simulink model "rtwdemo_paramdt"  (Simulink 7.6)
settings: Solver=FixedStepDiscrete  StartTime=0.0  StopTime=10.0  RelTol=1e-3  SampleTimeConstraint=STIndependent
PostLoadFcn:
  | rtwdemo_paramdt_data
undefined symbols (not defined in the file or in its folder): Kalias, Kcs, Kfixpt, Kinline, Kint8, Ksingle, Kuser
libraries: rtwdemowidgets x3
Description:
  | Controlling the Data Types of Tunable Parameters
settings Model: Creator=The MathWorks Inc.  CovMetricSettings=d  ExtModeAutoUpdateStatusClock=off  TunableVars=Kcs,Kint8,Ksingle  TunableVarsStorageClass=ExportedGlobal,ExportedGlobal,ExportedGlobal  TunableVarsTypeQualifier=,,
settings DataIOCC: SaveOutput=off  SaveTime=off  SignalLoggingName=sigsOut
settings OptimizationCC: InlineParams=on  InlineInvariantSignals=on  StateBitsets=on  DataBitsets=on  UseTempVars=on  EfficientFloat2IntCast=on  EfficientMapNaN2IntZero=off
settings DebuggingCC: CheckExecutionContextPreStartOutputMsg=on  CheckExecutionContextRuntimeOutputMsg=on  SolverPrmCheckMsg=none  ParameterDowncastMsg=none  ParameterOverflowMsg=none  ParameterPrecisionLossMsg=none  StrictBusMsg=ErrorOnBusTreatedAsVector
settings HardwareCC: ProdIntDivRoundTo=Zero  ProdEndianess=LittleEndian  ProdHWDeviceType=Generic->32-bit Embedded Processor  TargetIntDivRoundTo=Zero  TargetEndianess=LittleEndian  TargetHWDeviceType=Generic->MATLAB Host Computer  ProdEqTarget=off
settings SFSimCC: SimParseCustomCode=off
settings RTWCC: TLCOptions=-p0  GenerateReport=on  RTWVerbose=off  ProcessScript=grt_make_rtw_hook  LaunchReport=on
settings CodeAppCC: ForceParamTrailComments=on
settings GRTTargetCC: TargetFcnLib=ansi_tfl_tmw.mat

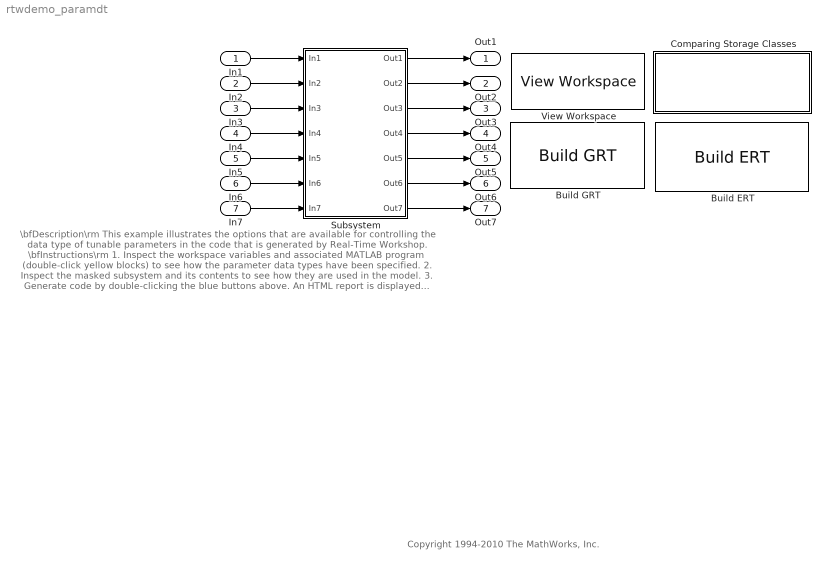
== system rtwdemo_paramdt ==
  note: \bfDescription\rm
      | This example illustrates the options that are available for controlling the data type of
      | tunable parameters in the code that is generated by Real-Time Workshop.
      |
      | \bfInstructions\rm
      | 1. Inspect the workspace variables and associated MATLAB program (double-click yellow blocks)
      |     to see how the parameter data types have been specified.
      | 2. Inspect the masked subsystem and its contents to see how they are used in the model.
      | 3. Generate code by double-clicking the blue buttons above.
      |     An HTML report is displayed automatically.
      | 4. Inspect the generated source files and take note of
      |     - The data types used in the parameter declarations/definitions
      |     - How the parameters are used in the code for the Gain and Saturation blocks
      |
      | \bfNote\rm
      | Inline parameters and storage classes must be selected to preserve parameter
      | identifiers in the generated code.
  note: Copyright 1994-2010 The MathWorks, Inc.
  In1 : Inport  OutDataTypeStr=single  PortDimensions=1
  In2 : Inport  Port=2  OutDataTypeStr=single  PortDimensions=1
  In3 : Inport  Port=3  OutDataTypeStr=single  PortDimensions=1
  In4 : Inport  Port=4  OutDataTypeStr=single  PortDimensions=1
  In5 : Inport  Port=5  OutDataTypeStr=single  PortDimensions=1
  In6 : Inport  Port=6  OutDataTypeStr=single  PortDimensions=1
  In7 : Inport  Port=7  OutDataTypeStr=single  PortDimensions=1
  Build ERT : rtwdemowidgets/Build ERT  SystemSampleTime=-1  attrib_overrides={}
  Build GRT : rtwdemowidgets/Build GRT  SystemSampleTime=-1  attrib_overrides={}
  Comparing Storage Classes : Subsystem
      settings: OpenFcn=edit rtwdemo_paramdt_data.m
      mask Display: disp(['View MATLAB program For\nCreating Variables\n(double-click)']);
  Subsystem : Subsystem
  View Workspace : rtwdemowidgets/View Workspace  SystemSampleTime=-1
  Out1 : Outport
  Out2 : Outport  Port=2
  Out3 : Outport  Port=3
  Out4 : Outport  Port=4
  Out5 : Outport  Port=5
  Out6 : Outport  Port=6
  Out7 : Outport  Port=7
  wires:
  In1/1 -> Subsystem/1(In1)
  In2/1 -> Subsystem/2(In2)
  In3/1 -> Subsystem/3(In3)
  In4/1 -> Subsystem/4(In4)
  In5/1 -> Subsystem/5(In5)
  In6/1 -> Subsystem/6(In6)
  In7/1 -> Subsystem/7(In7)
  Subsystem/1(Out1) -> Out1/1
  Subsystem/2(Out2) -> Out2/1
  Subsystem/3(Out3) -> Out3/1
  Subsystem/4(Out4) -> Out4/1
  Subsystem/5(Out5) -> Out5/1
  Subsystem/6(Out6) -> Out6/1
  Subsystem/7(Out7) -> Out7/1

== system rtwdemo_paramdt/Comparing Storage Classes ==

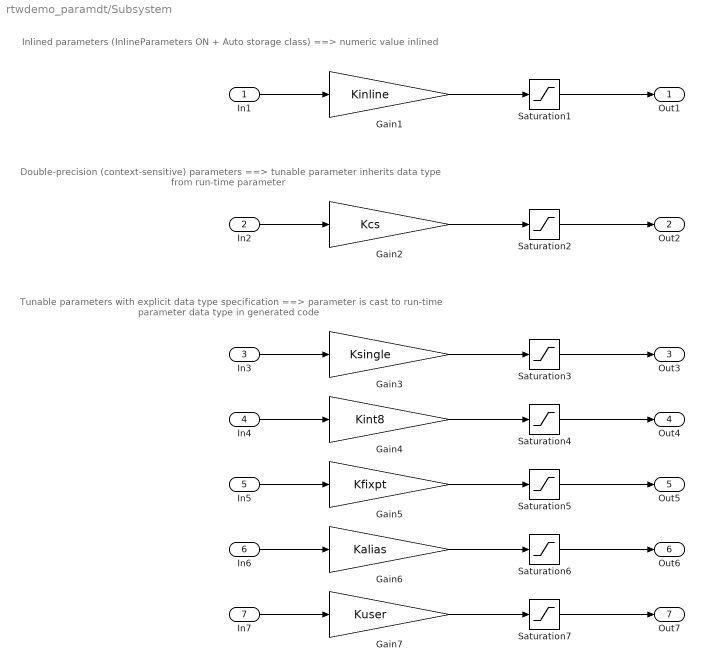
== system rtwdemo_paramdt/Subsystem ==
  note: Double-precision (context-sensitive) parameters
      | ==> tunable parameter inherits data type from run-time parameter
  note: Tunable parameters with explicit data type specification
      | ==> parameter is cast to run-time parameter data type in generated code
  note: Inlined parameters (InlineParameters ON + Auto storage class)
      | ==> numeric value inlined
  In1 : Inport  OutDataTypeStr=single
  In2 : Inport  Port=2  OutDataTypeStr=single
  In3 : Inport  Port=3  OutDataTypeStr=single
  In4 : Inport  Port=4  OutDataTypeStr=single
  In5 : Inport  Port=5  OutDataTypeStr=single
  In6 : Inport  Port=6  OutDataTypeStr=single
  In7 : Inport  Port=7  OutDataTypeStr=single
  Gain1 : Gain  Gain=Kinline  OutDataTypeStr=Inherit: Same as input  ParamDataTypeStr=Inherit: Same as input
  Gain2 : Gain  Gain=Kcs  OutDataTypeStr=Inherit: Same as input  ParamDataTypeStr=Inherit: Same as input
  Gain3 : Gain  Gain=Ksingle  OutDataTypeStr=Inherit: Same as input  ParamDataTypeStr=Inherit: Same as input
  Gain4 : Gain  Gain=Kint8  OutDataTypeStr=Inherit: Same as input  ParamDataTypeStr=Inherit: Same as input
  Gain5 : Gain  Gain=Kfixpt  OutDataTypeStr=Inherit: Same as input  ParamDataTypeStr=Inherit: Same as input
  Gain6 : Gain  Gain=Kalias  OutDataTypeStr=Inherit: Same as input  ParamDataTypeStr=Inherit: Same as input
  Gain7 : Gain  Gain=Kuser  OutDataTypeStr=Inherit: Same as input  ParamDataTypeStr=Inherit: Same as input
  Saturation1 : Saturate  UpperLimit=Kinline  LowerLimit=0
      settings: AttributesFormatString=Upper: %<UpperLimit>\nLower: %<LowerLimit>
  Saturation2 : Saturate  UpperLimit=Kcs  LowerLimit=0
      settings: AttributesFormatString=Upper: %<UpperLimit>\nLower: %<LowerLimit>
  Saturation3 : Saturate  UpperLimit=Ksingle  LowerLimit=0
      settings: AttributesFormatString=Upper: %<UpperLimit>\nLower: %<LowerLimit>
  Saturation4 : Saturate  UpperLimit=Kint8  LowerLimit=0
      settings: AttributesFormatString=Upper: %<UpperLimit>\nLower: %<LowerLimit>
  Saturation5 : Saturate  UpperLimit=Kfixpt  LowerLimit=0
      settings: AttributesFormatString=Upper: %<UpperLimit>\nLower: %<LowerLimit>
  Saturation6 : Saturate  UpperLimit=Kalias  LowerLimit=0
      settings: AttributesFormatString=Upper: %<UpperLimit>\nLower: %<LowerLimit>
  Saturation7 : Saturate  UpperLimit=Kuser  LowerLimit=0
      settings: AttributesFormatString=Upper: %<UpperLimit>\nLower: %<LowerLimit>
  Out1 : Outport
  Out2 : Outport  Port=2
  Out3 : Outport  Port=3
  Out4 : Outport  Port=4
  Out5 : Outport  Port=5
  Out6 : Outport  Port=6
  Out7 : Outport  Port=7
  wires:
  In2/1 -> Gain2/1
  Gain2/1 -> Saturation2/1
  In3/1 -> Gain3/1
  Gain3/1 -> Saturation3/1
  In4/1 -> Gain4/1
  Gain4/1 -> Saturation4/1
  In5/1 -> Gain5/1
  Gain5/1 -> Saturation5/1
  Saturation2/1 -> Out2/1
  Saturation3/1 -> Out3/1
  Saturation4/1 -> Out4/1
  Saturation5/1 -> Out5/1
  In6/1 -> Gain6/1
  Gain6/1 -> Saturation6/1
  Saturation6/1 -> Out6/1
  In7/1 -> Gain7/1
  Gain7/1 -> Saturation7/1
  Saturation7/1 -> Out7/1
  In1/1 -> Gain1/1
  Gain1/1 -> Saturation1/1
  Saturation1/1 -> Out1/1
